simulink model "hinf_control_with_integrator_multimodel_closed_loop_system"  (R2020b)
settings: Solver=VariableStepAuto  StartTime=0.0  StopTime=200  RelTol=1e-3
values from neighbouring files (symbols this model uses):
  COMMANDED_TORQUE_SATURATION = 0.05    [Workshop_MATLAB.m]
  COUPLING_COEFFICIENT = 0.5736    [Workshop_MATLAB.m]
  DISTURBANCE_TORQUE = 0.001    [Workshop_MATLAB.m]
  DISTURBANCE_TORQUE_DELAY = 100    [Workshop_MATLAB.m]
  ESTIMATOR_TRANSFER_FUNCTION_DENOMINATOR = [ESTIMATOR_TIME_CONSTANT 1]    [Workshop_MATLAB.m]
  ESTIMATOR_TRANSFER_FUNCTION_NUMERATOR = [1 0]    [Workshop_MATLAB.m]
  FLEXIBLE_MODE_DAMPING_RATIO = 0.00495    [Workshop_MATLAB.m]
  FLEXIBLE_MODE_FREQUENCY = 2.6268    [Workshop_MATLAB.m]
  INITIAL_CONDITION_ON_STATE = 0.0001    [Workshop_MATLAB.m]
  MAXIMUM_TOLERABLE_POINTING_ERROR = 3.5*2*pi/360    (= 0.0610865238198)    [Workshop_MATLAB.m]
  MEASUREMENT_NOISE_VARIANCE = 10^(-9)    (= 1e-09)    [Workshop_MATLAB.m]
  REACTION_WHEEL_DYNAMICS_DENOMINATOR = [1 2.400 0.763]    [Workshop_MATLAB.m]
  REACTION_WHEEL_DYNAMICS_NUMERATOR = REACTION_WHEEL_INERTIA*[1.214 0.763 0]    [Workshop_MATLAB.m]
  REACTION_WHEEL_INERTIA = 0.0004    [Workshop_MATLAB.m]
  REACTION_WHEEL_VELOCITY_SATURATION = 2800*2*pi/60    (= 293.215314335)    [Workshop_MATLAB.m]
  SATELLITE_INERTIA = 31.38    [Workshop_MATLAB.m]
  STAR_TRACKER_NOISE_DELAY = 160    [Workshop_MATLAB.m]
undefined symbols (not defined in the file or in its folder): hinfControlWithIntegratorMultimodelStateSpace, satelliteInertiaMaxWorstCase, satelliteInertiaMinWorstCase, TARGET_SECOND_ORDER
settings Model: Creator=WLCG  LastModifiedBy=WLCG

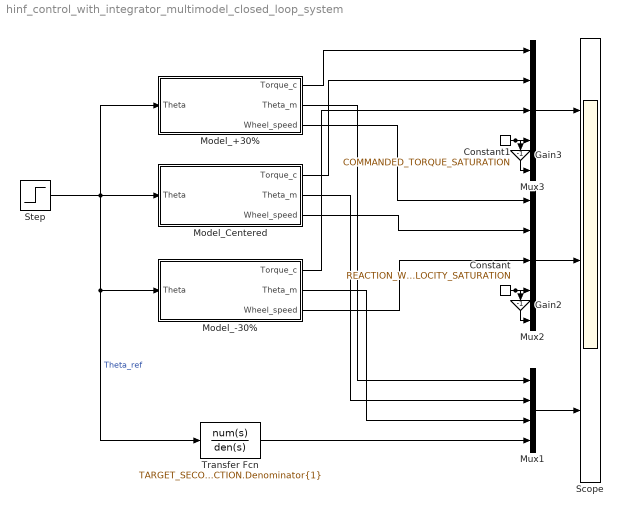
== system hinf_control_with_integrator_multimodel_closed_loop_system ==
  Constant : Constant  Value=REACTION_WHEEL_VELOCITY_SATURATION
  Constant1 : Constant  Value=COMMANDED_TORQUE_SATURATION
  Gain2 : Gain  Gain=-1
  Gain3 : Gain  Gain=-1
  Model_+30% : Subsystem
  Model_-30% : Subsystem
  Model_Centered : Subsystem
  Mux1 : Mux
  Mux2 : Mux  Inputs=5
  Mux3 : Mux  Inputs=5
  Scope : Scope  NumInputPorts=3
  Step : Step  Time=0  After=MAXIMUM_TOLERABLE_POINTING_ERROR  SampleTime=0
  Transfer Fcn : TransferFcn  Numerator=TARGET_SECOND_ORDER.TRANSFER_FUNCTION.Numerator{1}  Denominator=TARGET_SECOND_ORDER.TRANSFER_FUNCTION.Denominator{1}
  wires:
  Step/1 -> Model_-30%/1(Theta), Transfer Fcn/1, Model_Centered/1(Theta), Model_+30%/1(Theta)  "Theta_ref"
  Transfer Fcn/1 -> Mux1/4
  Model_Centered/2(Theta_m) -> Mux1/2
  Model_+30%/2(Theta_m) -> Mux1/1
  Model_-30%/2(Theta_m) -> Mux1/3
  Mux1/1 -> Scope/3
  Mux2/1 -> Scope/2
  Model_-30%/3(Wheel_speed) -> Mux2/3
  Model_Centered/3(Wheel_speed) -> Mux2/2
  Model_+30%/3(Wheel_speed) -> Mux2/1
  Mux3/1 -> Scope/1
  Model_-30%/1(Torque_c) -> Mux3/3
  Model_Centered/1(Torque_c) -> Mux3/2
  Model_+30%/1(Torque_c) -> Mux3/1
  Constant1/1 -> Gain3/1, Mux3/4
  Gain3/1 -> Mux3/5
  Constant/1 -> Gain2/1, Mux2/4
  Gain2/1 -> Mux2/5

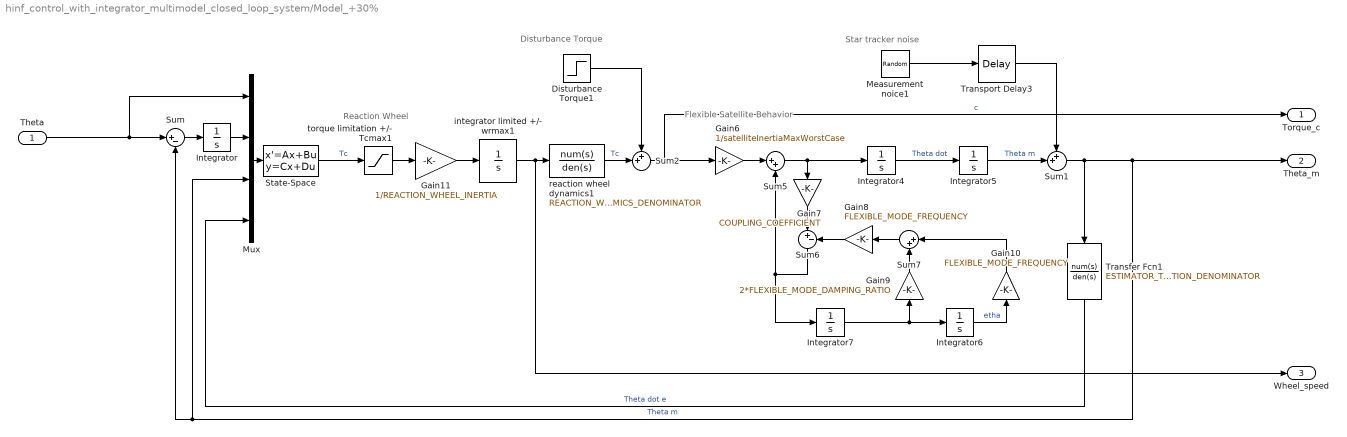
== system hinf_control_with_integrator_multimodel_closed_loop_system/Model_+30% ==
  note: Star tracker noise
  note: Flexible Satellite Behavior
  note: Disturbance Torque
  note: Reaction Wheel
  Theta : Inport
  Disturbance Torque1 : Step  Time=DISTURBANCE_TORQUE_DELAY  After=DISTURBANCE_TORQUE  SampleTime=0
  Gain10 : Gain  Gain=FLEXIBLE_MODE_FREQUENCY
  Gain11 : Gain  Gain=1/REACTION_WHEEL_INERTIA
  Gain6 : Gain  Gain=1/satelliteInertiaMaxWorstCase
  Gain7 : Gain  Gain=COUPLING_COEFFICIENT
  Gain8 : Gain  Gain=FLEXIBLE_MODE_FREQUENCY
  Gain9 : Gain  Gain=2*FLEXIBLE_MODE_DAMPING_RATIO
  Integrator{,4..5,7} (4 alike) : Integrator
  Integrator6 : Integrator  InitialCondition=INITIAL_CONDITION_ON_STATE
  Measurement noice1 : RandomNumber  Variance=MEASUREMENT_NOISE_VARIANCE  SampleTime=0.01
  Mux : Mux
  State-Space : StateSpace  A=hinfControlWithIntegratorMultimodelStateSpace.A  B=hinfControlWithIntegratorMultimodelStateSpace.B  C=hinfControlWithIntegratorMultimodelStateSpace.C  D=hinfControlWithIntegratorMultimodelStateSpace.D  InitialCondition=0
  Sum : Sum  Inputs=|+-
  Sum1 : Sum  Inputs=++|
  Sum2 : Sum  Inputs=++|
  Sum5 : Sum  Inputs=|++
  Sum6 : Sum  Inputs=|+-
  Sum7 : Sum  Inputs=|++
  Transfer Fcn1 : TransferFcn  Numerator=ESTIMATOR_TRANSFER_FUNCTION_NUMERATOR  Denominator=ESTIMATOR_TRANSFER_FUNCTION_DENOMINATOR
  Transport Delay3 : TransportDelay  DelayTime=STAR_TRACKER_NOISE_DELAY
  integrator limited +/- wrmax1 : Integrator  LimitOutput=on  UpperSaturationLimit=REACTION_WHEEL_VELOCITY_SATURATION  LowerSaturationLimit=-REACTION_WHEEL_VELOCITY_SATURATION
  reaction wheel dynamics1 : TransferFcn  Numerator=REACTION_WHEEL_DYNAMICS_NUMERATOR  Denominator=REACTION_WHEEL_DYNAMICS_DENOMINATOR
  torque limitation +/- Tcmax1 : Saturate  UpperLimit=COMMANDED_TORQUE_SATURATION  LowerLimit=-COMMANDED_TORQUE_SATURATION
  Torque_c : Outport
  Theta_m : Outport  Port=2
  Wheel_speed : Outport  Port=3
  wires:
  Transfer Fcn1/1 -> Mux/4  "Theta dot e"
  Sum1/1 -> Theta_m/1, Mux/3, Sum/2, Transfer Fcn1/1  "Theta m"
  Gain10/1 -> Sum7/1
  Gain8/1 -> Sum6/2
  Measurement noice1/1 -> Transport Delay3/1
  State-Space/1 -> torque limitation +/- Tcmax1/1  "Tc"
  Integrator/1 -> Mux/2
  Sum2/1 -> Torque_c/1, Gain6/1  "c"
  Integrator4/1 -> Integrator5/1  "Theta dot"
  Gain6/1 -> Sum5/1
  Disturbance Torque1/1 -> Sum2/1
  Transport Delay3/1 -> Sum1/1
  Sum6/1 -> Integrator7/1, Sum5/2
  Theta/1 -> Mux/1, Sum/1
  Mux/1 -> State-Space/1
  Gain9/1 -> Sum7/2
  Gain11/1 -> integrator limited +/- wrmax1/1
  torque limitation +/- Tcmax1/1 -> Gain11/1
  Integrator7/1 -> Integrator6/1, Gain9/1
  Integrator5/1 -> Sum1/2  "Theta m"
  Sum5/1 -> Integrator4/1, Gain7/1
  reaction wheel dynamics1/1 -> Sum2/2  "Tc"
  integrator limited +/- wrmax1/1 -> Wheel_speed/1, reaction wheel dynamics1/1
  Gain7/1 -> Sum6/1
  Integrator6/1 -> Gain10/1  "etha"
  Sum/1 -> Integrator/1
  Sum7/1 -> Gain8/1

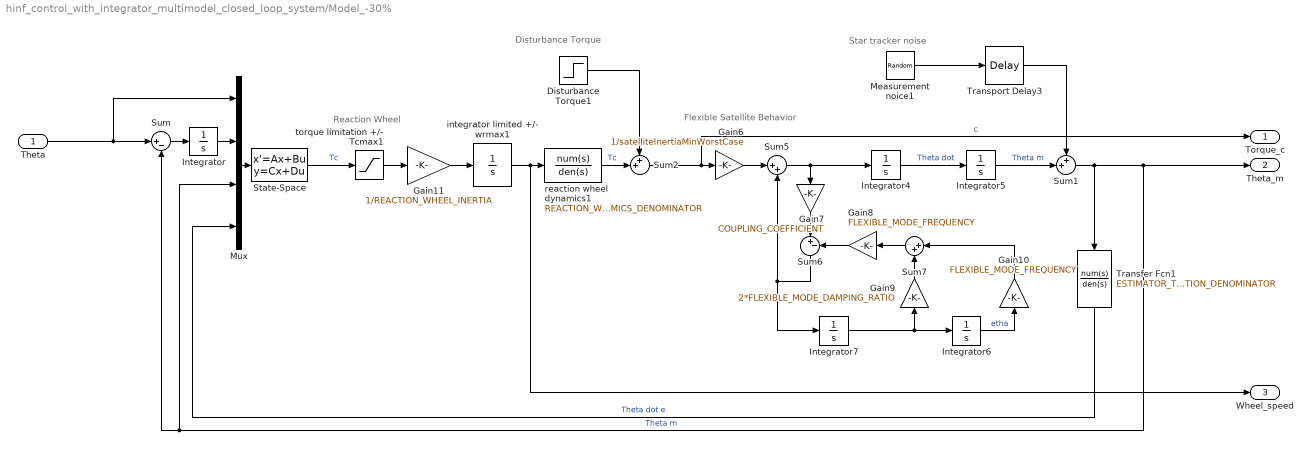
== system hinf_control_with_integrator_multimodel_closed_loop_system/Model_-30% ==
  note: Disturbance Torque
  note: Star tracker noise
  note: Flexible Satellite Behavior
  note: Reaction Wheel
  Theta : Inport
  Disturbance Torque1 : Step  Time=DISTURBANCE_TORQUE_DELAY  After=DISTURBANCE_TORQUE  SampleTime=0
  Gain10 : Gain  Gain=FLEXIBLE_MODE_FREQUENCY
  Gain11 : Gain  Gain=1/REACTION_WHEEL_INERTIA
  Gain6 : Gain  Gain=1/satelliteInertiaMinWorstCase
  Gain7 : Gain  Gain=COUPLING_COEFFICIENT
  Gain8 : Gain  Gain=FLEXIBLE_MODE_FREQUENCY
  Gain9 : Gain  Gain=2*FLEXIBLE_MODE_DAMPING_RATIO
  Integrator{,4..5,7} (4 alike) : Integrator
  Integrator6 : Integrator  InitialCondition=INITIAL_CONDITION_ON_STATE
  Measurement noice1 : RandomNumber  Variance=MEASUREMENT_NOISE_VARIANCE  SampleTime=0.01
  Mux : Mux
  State-Space : StateSpace  A=hinfControlWithIntegratorMultimodelStateSpace.A  B=hinfControlWithIntegratorMultimodelStateSpace.B  C=hinfControlWithIntegratorMultimodelStateSpace.C  D=hinfControlWithIntegratorMultimodelStateSpace.D  InitialCondition=0
  Sum : Sum  Inputs=|+-
  Sum1 : Sum  Inputs=++|
  Sum2 : Sum  Inputs=++|
  Sum5 : Sum  Inputs=|++
  Sum6 : Sum  Inputs=|+-
  Sum7 : Sum  Inputs=|++
  Transfer Fcn1 : TransferFcn  Numerator=ESTIMATOR_TRANSFER_FUNCTION_NUMERATOR  Denominator=ESTIMATOR_TRANSFER_FUNCTION_DENOMINATOR
  Transport Delay3 : TransportDelay  DelayTime=STAR_TRACKER_NOISE_DELAY
  integrator limited +/- wrmax1 : Integrator  LimitOutput=on  UpperSaturationLimit=REACTION_WHEEL_VELOCITY_SATURATION  LowerSaturationLimit=-REACTION_WHEEL_VELOCITY_SATURATION
  reaction wheel dynamics1 : TransferFcn  Numerator=REACTION_WHEEL_DYNAMICS_NUMERATOR  Denominator=REACTION_WHEEL_DYNAMICS_DENOMINATOR
  torque limitation +/- Tcmax1 : Saturate  UpperLimit=COMMANDED_TORQUE_SATURATION  LowerLimit=-COMMANDED_TORQUE_SATURATION
  Torque_c : Outport
  Theta_m : Outport  Port=2
  Wheel_speed : Outport  Port=3
  wires:
  Sum1/1 -> Mux/3, Sum/2, Theta_m/1, Transfer Fcn1/1  "Theta m"
  Gain9/1 -> Sum7/2
  Integrator4/1 -> Integrator5/1  "Theta dot"
  torque limitation +/- Tcmax1/1 -> Gain11/1
  Gain10/1 -> Sum7/1
  Sum7/1 -> Gain8/1
  Transfer Fcn1/1 -> Mux/4  "Theta dot e"
  integrator limited +/- wrmax1/1 -> Wheel_speed/1, reaction wheel dynamics1/1
  Sum/1 -> Integrator/1
  Integrator7/1 -> Integrator6/1, Gain9/1
  Gain6/1 -> Sum5/1
  Transport Delay3/1 -> Sum1/1
  Sum5/1 -> Integrator4/1, Gain7/1
  Mux/1 -> State-Space/1
  Disturbance Torque1/1 -> Sum2/1
  Sum6/1 -> Integrator7/1, Sum5/2
  Integrator6/1 -> Gain10/1  "etha"
  reaction wheel dynamics1/1 -> Sum2/2  "Tc"
  Gain7/1 -> Sum6/1
  State-Space/1 -> torque limitation +/- Tcmax1/1  "Tc"
  Measurement noice1/1 -> Transport Delay3/1
  Sum2/1 -> Torque_c/1, Gain6/1  "c"
  Gain8/1 -> Sum6/2
  Gain11/1 -> integrator limited +/- wrmax1/1
  Integrator5/1 -> Sum1/2  "Theta m"
  Integrator/1 -> Mux/2
  Theta/1 -> Sum/1, Mux/1

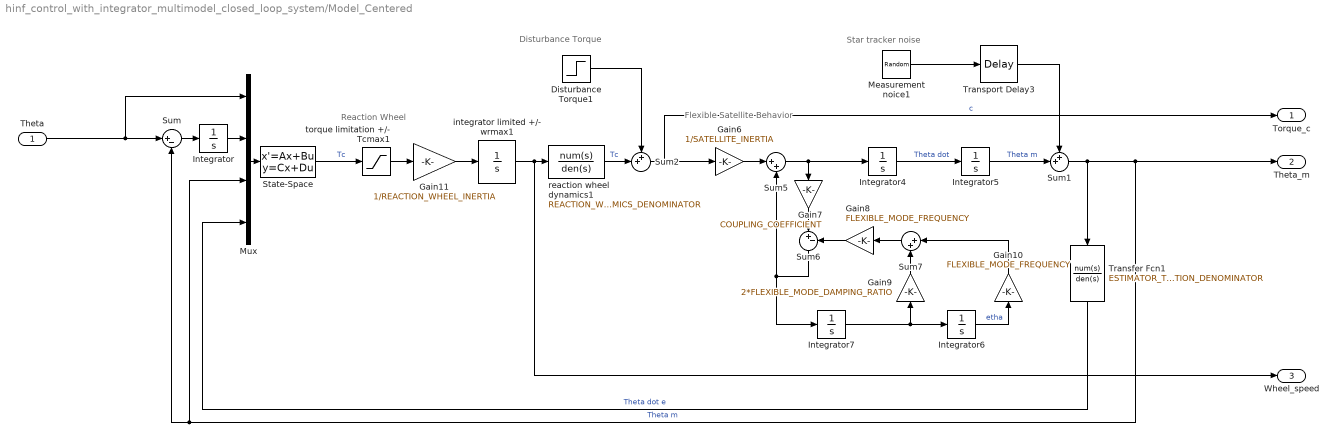
== system hinf_control_with_integrator_multimodel_closed_loop_system/Model_Centered ==
  note: Disturbance Torque
  note: Flexible Satellite Behavior
  note: Star tracker noise
  note: Reaction Wheel
  Theta : Inport
  Disturbance Torque1 : Step  Time=DISTURBANCE_TORQUE_DELAY  After=DISTURBANCE_TORQUE  SampleTime=0
  Gain10 : Gain  Gain=FLEXIBLE_MODE_FREQUENCY
  Gain11 : Gain  Gain=1/REACTION_WHEEL_INERTIA
  Gain6 : Gain  Gain=1/SATELLITE_INERTIA
  Gain7 : Gain  Gain=COUPLING_COEFFICIENT
  Gain8 : Gain  Gain=FLEXIBLE_MODE_FREQUENCY
  Gain9 : Gain  Gain=2*FLEXIBLE_MODE_DAMPING_RATIO
  Integrator{,4..5,7} (4 alike) : Integrator
  Integrator6 : Integrator  InitialCondition=INITIAL_CONDITION_ON_STATE
  Measurement noice1 : RandomNumber  Variance=MEASUREMENT_NOISE_VARIANCE  SampleTime=0.01
  Mux : Mux
  State-Space : StateSpace  A=hinfControlWithIntegratorMultimodelStateSpace.A  B=hinfControlWithIntegratorMultimodelStateSpace.B  C=hinfControlWithIntegratorMultimodelStateSpace.C  D=hinfControlWithIntegratorMultimodelStateSpace.D  InitialCondition=0
  Sum : Sum  Inputs=|+-
  Sum1 : Sum  Inputs=++|
  Sum2 : Sum  Inputs=++|
  Sum5 : Sum  Inputs=|++
  Sum6 : Sum  Inputs=|+-
  Sum7 : Sum  Inputs=|++
  Transfer Fcn1 : TransferFcn  Numerator=ESTIMATOR_TRANSFER_FUNCTION_NUMERATOR  Denominator=ESTIMATOR_TRANSFER_FUNCTION_DENOMINATOR
  Transport Delay3 : TransportDelay  DelayTime=STAR_TRACKER_NOISE_DELAY
  integrator limited +/- wrmax1 : Integrator  LimitOutput=on  UpperSaturationLimit=REACTION_WHEEL_VELOCITY_SATURATION  LowerSaturationLimit=-REACTION_WHEEL_VELOCITY_SATURATION
  reaction wheel dynamics1 : TransferFcn  Numerator=REACTION_WHEEL_DYNAMICS_NUMERATOR  Denominator=REACTION_WHEEL_DYNAMICS_DENOMINATOR
  torque limitation +/- Tcmax1 : Saturate  UpperLimit=COMMANDED_TORQUE_SATURATION  LowerLimit=-COMMANDED_TORQUE_SATURATION
  Torque_c : Outport
  Theta_m : Outport  Port=2
  Wheel_speed : Outport  Port=3
  wires:
  Transport Delay3/1 -> Sum1/1
  State-Space/1 -> torque limitation +/- Tcmax1/1  "Tc"
  Sum7/1 -> Gain8/1
  Sum2/1 -> Gain6/1, Torque_c/1  "c"
  Integrator7/1 -> Integrator6/1, Gain9/1
  Measurement noice1/1 -> Transport Delay3/1
  Gain7/1 -> Sum6/1
  Integrator6/1 -> Gain10/1  "etha"
  Sum/1 -> Integrator/1
  integrator limited +/- wrmax1/1 -> Wheel_speed/1, reaction wheel dynamics1/1
  Theta/1 -> Mux/1, Sum/1
  Sum5/1 -> Integrator4/1, Gain7/1
  reaction wheel dynamics1/1 -> Sum2/2  "Tc"
  Mux/1 -> State-Space/1
  Disturbance Torque1/1 -> Sum2/1
  Sum6/1 -> Integrator7/1, Sum5/2
  Integrator/1 -> Mux/2
  Gain6/1 -> Sum5/1
  Transfer Fcn1/1 -> Mux/4  "Theta dot e"
  Integrator4/1 -> Integrator5/1  "Theta dot"
  Gain10/1 -> Sum7/1
  Sum1/1 -> Mux/3, Sum/2, Theta_m/1, Transfer Fcn1/1  "Theta m"
  torque limitation +/- Tcmax1/1 -> Gain11/1
  Gain11/1 -> integrator limited +/- wrmax1/1
  Integrator5/1 -> Sum1/2  "Theta m"
  Gain9/1 -> Sum7/2
  Gain8/1 -> Sum6/2
